simulink model "coupled_pendulum"  (R2016a)
settings: Solver=ode23  StartTime=0.0  StopTime=tfinal  MaxStep=0.01  RelTol=1e-3
values from neighbouring files (symbols this model uses):
  cd = 0.05    [runSimulink_single_pendulum.m]
  g = 9.8    [runSimulink_single_pendulum.m]
  m = 1.5    [runSimulink_single_pendulum.m]
  thetaA_0 = pi/8    (= 0.392699081699)    [runSimulink_single_pendulum.m]
undefined symbols (not defined in the file or in its folder): k, l1, l2
settings Model: Creator=dqtm  LastModifiedBy=dqtm
settings DataIOCC: LimitDataPoints=on  SaveFormat=Array  SignalLoggingSaveFormat=ModelDataLogs
settings OptimizationCC: ExpressionDepthLimit=2147483647  InitFltsAndDblsToZero=on
settings DebuggingCC: UnderspecifiedInitializationDetection=Classic  MergeDetectMultiDrivingBlocksExec=none  SolverPrmCheckMsg=warning  FcnCallInpInsideContextMsg=UseLocalSettings  StateNameClashWarn=warning  StrictBusMsg=Warning
settings HardwareCC: ProdBitPerPointer=32  ProdLargestAtomicFloat=None  ProdIntDivRoundTo=Undefined  ProdEndianess=Unspecified  ProdWordSize=32  ProdHWDeviceType=32-bit Generic
settings ModelReferenceCC: PropagateSignalLabelsOutOfModel=off
settings GRTTargetCC: CombineOutputUpdateFcns=off  GRTInterface=on
settings ConfigComp: CovModelRefEnable=Off

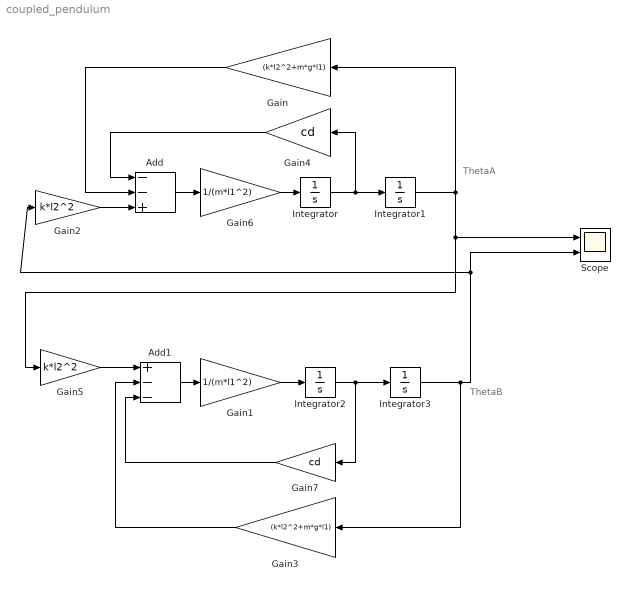
== system coupled_pendulum ==
  note: ThetaA
  note: ThetaB
  Add : Sum  Inputs=--+
  Add1 : Sum  Inputs=+--
  Gain : Gain  Gain=(k*l2^2+m*g*l1)
  Gain1 : Gain  Gain=1/(m*l1^2)
  Gain2 : Gain  Gain=k*l2^2
  Gain3 : Gain  Gain=(k*l2^2+m*g*l1)
  Gain4 : Gain  Gain=cd
  Gain5 : Gain  Gain=k*l2^2
  Gain6 : Gain  Gain=1/(m*l1^2)
  Gain7 : Gain  Gain=cd
  Integrator : Integrator
  Integrator1 : Integrator  InitialCondition=thetaA_0
  Integrator2 : Integrator
  Integrator3 : Integrator
  Scope : Scope  NumInputPorts=2
  wires:
  Integrator/1 -> Integrator1/1, Gain4/1
  Add/1 -> Gain6/1
  Integrator1/1 -> Gain/1, Gain5/1, Scope/1
  Integrator2/1 -> Integrator3/1, Gain7/1
  Add1/1 -> Gain1/1
  Integrator3/1 -> Gain2/1, Scope/2, Gain3/1
  Gain5/1 -> Add1/1
  Gain6/1 -> Integrator/1
  Gain3/1 -> Add1/2
  Gain1/1 -> Integrator2/1
  Gain2/1 -> Add/3
  Gain/1 -> Add/2
  Gain4/1 -> Add/1
  Gain7/1 -> Add1/3
